simulink model "Motor_Speed_to_Commands"  (R2020a)
settings: Solver=VariableStepAuto  StartTime=0.0  StopTime=10.0  RelTol=1e-3
undefined symbols (not defined in the file): b, k, l
settings Model: Creator=prans  LastModifiedBy=prans

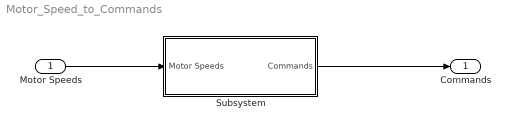
== system Motor_Speed_to_Commands ==
  Motor Speeds : Inport
  Subsystem : Subsystem
  Commands : Outport
  wires:
  Motor Speeds/1 -> Subsystem/1(Motor Speeds)
  Subsystem/1(Commands) -> Commands/1

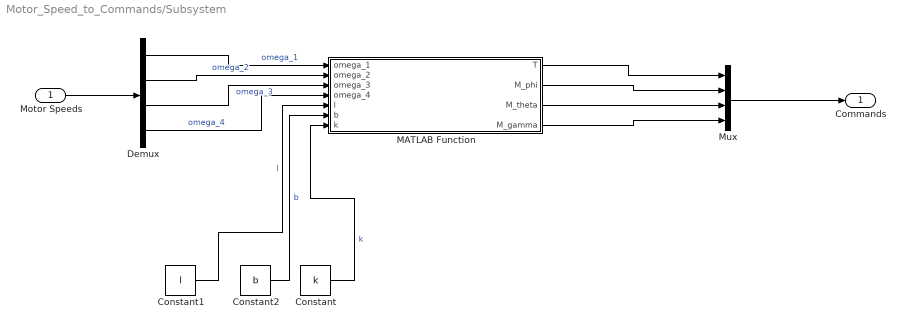
== system Motor_Speed_to_Commands/Subsystem ==
  Motor Speeds : Inport
  Constant : Constant  Value=k
  Constant1 : Constant  Value=l
  Constant2 : Constant  Value=b
  Demux : Demux
  MATLAB Function : MATLAB Function  TreatAsAtomicUnit=on
  Mux : Mux
  Commands : Outport
  wires:
  Constant2/1 -> MATLAB Function/6(b)  "b"
  Demux/2 -> MATLAB Function/2(omega_2)  "omega_2"
  Constant/1 -> MATLAB Function/7(k)  "k"
  MATLAB Function/4(M_gamma) -> Mux/4
  Constant1/1 -> MATLAB Function/5(l)  "l"
  MATLAB Function/3(M_theta) -> Mux/3
  MATLAB Function/1(T) -> Mux/1
  MATLAB Function/2(M_phi) -> Mux/2
  Demux/3 -> MATLAB Function/3(omega_3)  "omega_3"
  Demux/1 -> MATLAB Function/1(omega_1)  "omega_1"
  Demux/4 -> MATLAB Function/4(omega_4)  "omega_4"
  Mux/1 -> Commands/1
  Motor Speeds/1 -> Demux/1

== matlab function Motor_Speed_to_Commands/Subsystem/MATLAB Function ==
  data: omega_1 input; T output; omega_2 input; omega_3 input; omega_4 input; l input; b input; k input; M_phi output; M_theta output; M_gamma output
function [T,M_phi,M_theta,M_gamma] = fcn(omega_1, omega_2, omega_3, omega_4, l, b, k)

omega_1 = omega_1^2;
omega_2 = omega_2^2;
omega_3 = omega_3^2;
omega_4 = omega_4^2;

T = k(omega_1+omega_2+omega_3+omega_4);
M_phi = k*l*omega_2 - k*l*omega_4;
M_theta = -k*l*omega_1 + k*l*omega_3;
M_gamma = b*(-omega_1 + omega_2 - omega_3 + omega_4);
